simulink model "Test3"  (R2014a)
settings: Solver=FixedStepDiscrete  SolverMode=SingleTasking  StartTime=0.0  StopTime=inf  FixedStep=0.01  RelTol=1e-3
undefined symbols (not defined in the file or in its folder): dacNum
libraries: EEE481Arduino x3
settings Model: SimulationMode=external  ExtModeTrigDuration=2  Creator=rsjoshi1  LastModifiedBy=rsjoshi1
settings OptimizationCC: OptimizeModelRefInitCode=on  LifeSpan=1
settings DebuggingCC: UnderspecifiedInitializationDetection=Classic  SolverPrmCheckMsg=none
settings HardwareCC: ProdLargestAtomicInteger=Long  ProdLargestAtomicFloat=Double  ProdEndianess=LittleEndian  ProdHWDeviceType=ARM Compatible->ARM Cortex
settings RTWCC: SystemTargetFile=realtime.tlc  GenerateMakefile=off  TemplateMakefile=realtime.tmf  Description=Run on Target Hardware  RTWVerbose=off  ProcessScript=realtime_make_rtw_hook
settings STFCustomTargetCC: TargetLibSuffix=.a  GenerateSampleERTMain=on  ConcurrentExecutionCompliant=off  GeneratePreprocessorConditionals=Use local settings  ERTCustomFileBanners=on  SupportNonInlinedSFcns=off  SupportVariableSizeSignals=on  MATLABClassNameForMDSCustomization=Simulink.SoftwareTarget.ERTCustomization  GRTInterface=off  SystemTargetFile=realtime.tlc
settings ERTTargetCC: CombineOutputUpdateFcns=off  SupportContinuousTime=on  SupportVariableSizeSignals=on  ExtModeTransport=3  ExtModeMexFile=ext_serial_win32_comm  ExtModeMexArgs=0 1 9600  ERTSrcFileBannerTemplate=realtime_code_template.cgt  ERTHdrFileBannerTemplate=realtime_code_template.cgt  ERTDataSrcFileTemplate=realtime_code_template.cgt  ERTDataHdrFileTemplate=realtime_code_template.cgt  ERTCustomFileTemplate=realtime_file_process.tlc

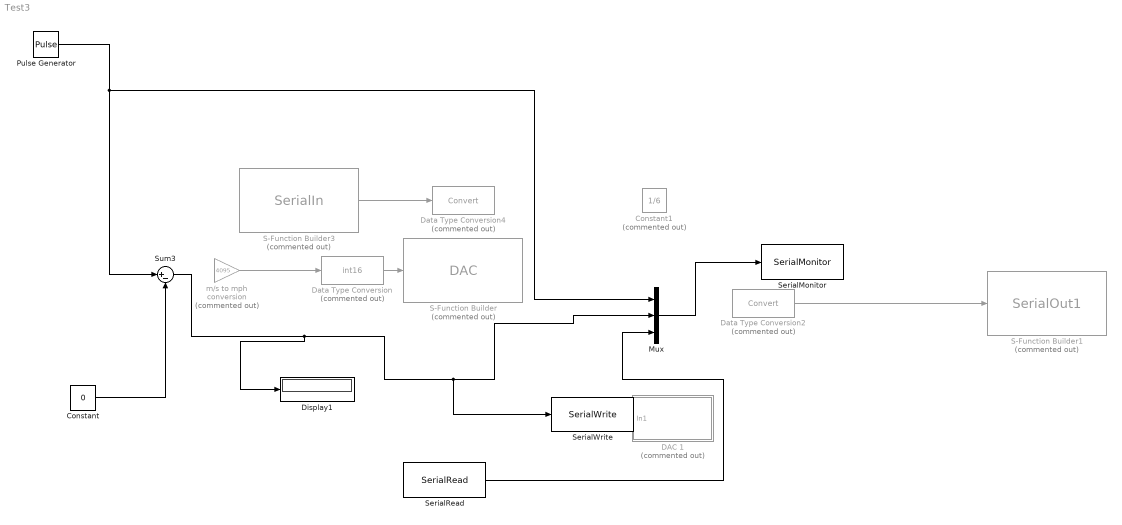
== system Test3 ==
  Constant : Constant  Value=0
  Constant1 : Constant  Commented=on  Value=1/6
  DAC 1 : Subsystem  Commented=on  mask{Tsa=-1, dacNum=1}
      mask prompts: Tsa "Sampling Time"; dacNum "DAC number(0 or 1)"
  Data Type Conversion : DataTypeConversion  Commented=on  OutDataTypeStr=int16
  Data Type Conversion2 : DataTypeConversion  Commented=on
  Data Type Conversion4 : DataTypeConversion  Commented=on
  Display1 : Display
  Mux : Mux  Inputs=3
  Pulse Generator : DiscretePulseGenerator  PulseType=Time based  Amplitude=5  Period=10  PulseWidth=90
  S-Function Builder : S-Function  Commented=on  InitFcn=try, set_param(gcb,'FunctionName','DAC'), end  FunctionName=DAC  Parameters=int8(dacNum)  SFunctionModules=DAC_wrapper  EnableBusSupport=off  mask(S-Function Builder){}
      mask help: Simulink:masks:SFunctionBuilder_MD
      mask init:
      | val = [[.9  0.75 0.75 1 1 .9 .9 1]',[1 1 0.75 0.75 .9 .9 1 .9]'];try , sys = get_param(gcb,'SfunBuilderFcnName');if isempty(sys), sys = get_param(gcb,'FunctionName'); end,catch, sys = get_param(gcb,'FunctionName'); end
      settings: CopyFcn=set_param(gcbh,'LinkStatus','none')  PreSaveFcn=try, set_param(gcb,'FunctionName','DAC'), end  OpenFcn=sfunctionwizard(gcbh)
      mask Display: plot(val(:,1),val(:,2)),disp(sys), port_label('input',1,'input')
  S-Function Builder1 : S-Function  Commented=on  InitFcn=try, set_param(gcb,'FunctionName','SerialOut1'), end  FunctionName=SerialOut1  Parameters=int8(0)  SFunctionModules=SerialOut1_wrapper  EnableBusSupport=off  mask(S-Function Builder){}
      mask help: Simulink:masks:SFunctionBuilder_MD
      mask init: same as Test3/S-Function Builder
      settings: CopyFcn=set_param(gcbh,'LinkStatus','none')  PreSaveFcn=try, set_param(gcb,'FunctionName','SerialOut1'), end  OpenFcn=sfunctionwizard(gcbh)
      mask Display: plot(val(:,1),val(:,2)),disp(sys), port_label('input',1,'input')
  S-Function Builder3 : S-Function  Commented=on  InitFcn=try, set_param(gcb,'FunctionName','SerialIn'), end  FunctionName=SerialIn  Parameters=int8(0)  SFunctionModules=SerialIn_wrapper  EnableBusSupport=off  mask(S-Function Builder){}
      mask help: Simulink:masks:SFunctionBuilder_MD
      mask init: same as Test3/S-Function Builder
      settings: CopyFcn=set_param(gcbh,'LinkStatus','none')  PreSaveFcn=try, set_param(gcb,'FunctionName','SerialIn'), end  OpenFcn=sfunctionwizard(gcbh)
      mask Display: plot(val(:,1),val(:,2)),disp(sys), port_label('output',1,'Out')
  SerialMonitor : EEE481Arduino/SerialMonitor  SystemSampleTime=-1
  SerialRead : EEE481Arduino/SerialRead  serialNum=2
  SerialWrite : EEE481Arduino/SerialWrite  serialNum=2
  Sum3 : Sum  Inputs=|+-
  m/s to mph conversion : Gain  Commented=on  Gain=4095  SaturateOnIntegerOverflow=on  OutDataTypeStr=Inherit: Same as input  ParamDataTypeStr=Inherit: Same as input
  wires:
  Data Type Conversion/1 -> S-Function Builder/1
  m/s to mph conversion/1 -> Data Type Conversion/1
  Constant/1 -> Sum3/2
  Pulse Generator/1 -> Mux/1, Sum3/1
  Data Type Conversion2/1 -> S-Function Builder1/1
  Mux/1 -> SerialMonitor/1
  Sum3/1 -> Display1/1, SerialWrite/1, Mux/2
  S-Function Builder3/1 -> Data Type Conversion4/1
  SerialRead/1 -> Mux/3

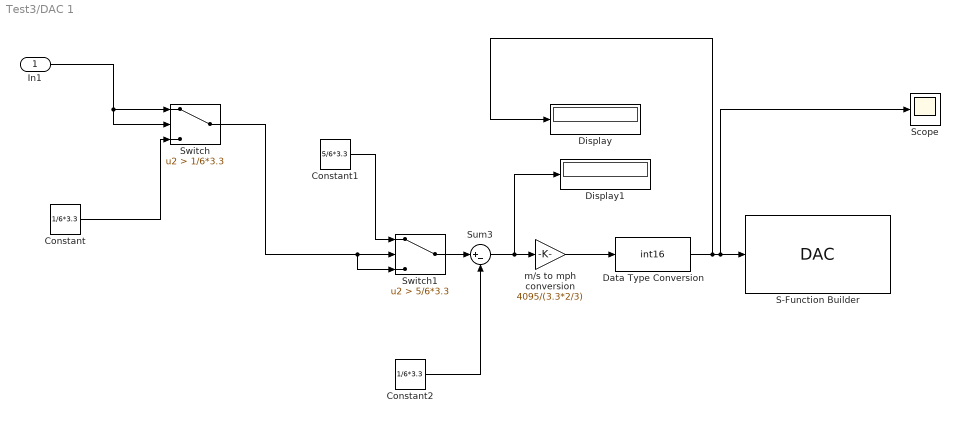
== system Test3/DAC 1 ==
  In1 : Inport  SampleTime=Tsa
  Constant : Constant  Value=1/6*3.3
  Constant1 : Constant  Value=5/6*3.3
  Constant2 : Constant  Value=1/6*3.3
  Data Type Conversion : DataTypeConversion  OutDataTypeStr=int16
  Display : Display
  Display1 : Display
  S-Function Builder : S-Function  InitFcn=try, set_param(gcb,'FunctionName','DAC'), end  FunctionName=DAC  Parameters=int8(dacNum)  SFunctionModules=DAC_wrapper  EnableBusSupport=off  mask(S-Function Builder){}
      mask help: Simulink:masks:SFunctionBuilder_MD
      mask init: same as Test3/S-Function Builder
      settings: CopyFcn=set_param(gcbh,'LinkStatus','none')  PreSaveFcn=try, set_param(gcb,'FunctionName','DAC'), end  OpenFcn=sfunctionwizard(gcbh)
      mask Display: plot(val(:,1),val(:,2)),disp(sys), port_label('input',1,'input')
  Scope : Scope
      settings: YMin=3890.25  YMax=4299.75  SaveName=ScopeData2
  Sum3 : Sum  Inputs=|+-
  Switch : Switch  Criteria=u2 > Threshold  Threshold=1/6*3.3
  Switch1 : Switch  Criteria=u2 > Threshold  Threshold=5/6*3.3
  m/s to mph conversion : Gain  Gain=4095/(3.3*2/3)  SaturateOnIntegerOverflow=on  OutDataTypeStr=Inherit: Same as input  ParamDataTypeStr=Inherit: Same as input
  wires:
  Constant2/1 -> Sum3/2
  Sum3/1 -> m/s to mph conversion/1, Display1/1
  Switch1/1 -> Sum3/1
  Constant1/1 -> Switch1/1
  Switch/1 -> Switch1/2, Switch1/3
  Constant/1 -> Switch/3
  In1/1 -> Switch/1, Switch/2
  m/s to mph conversion/1 -> Data Type Conversion/1
  Data Type Conversion/1 -> S-Function Builder/1, Scope/1, Display/1
